simulink model "MicroADAPCPU1"  (R2024a)
settings: Solver=FixedStepAuto  StartTime=0.0  StopTime=Inf  RelTol=1e-3  EnableMultiTasking=on
PreLoadFcn:
  | %Condiciones iniciales
  | id0=single(0);
  | iq0=single(0);
  | w0=single(0);
  | Thetha0=single(0);
  | deltars=0;
  | deltaLd=0;
  | deltaLq=0;
  | deltaphi=0;
  | 
  | %Parametros Axel;
  | Rs=single(1.1); %Ohms
  | L=single(0.00372);
  | Ld=L; %Henrry
  | Lq=L; %Henrry
  | Jm=single(0.00023998); %Kg m2
  | Rm=single(0.0006738); %Nm s
  | rm=Rm;
  | phi=single(0.1099); %Wb
  | %0.0582
  | np=single(8);
values from neighbouring files (symbols this model uses):
  target = mcb_SetProcessorDetails('F28379D',PWM_frequency)    [Para_Motor_Micro.m]
  Ts_com = 2*1*Ts    (= 6e-05)    [Para_Motor_Micro.m]
undefined symbols (not defined in the file or in its folder): C28x, CPU1, CPU2, DiscIntNeverNeededParam, Down, GPTRIP1SEL, GPTRIP2SEL, inverter, PWM_Counter_PeriodVel, TZ1, TZ2, Up
libraries: c2802xlib x12, mcbcontrolslib x9, c2837xDlib x8, simulink x4, mcbpositiondecoderlib x3, c280xlib x3, svdutilitieslib x2, eeTransforms x1, c2000lib x1
(part 2 of 2)

== system MicroADAPCPU1/Comms/SCI (Code Generation) 40khz/While Iterator Subsystem ==
  Data : Inport
  Iteration : Inport  Port=2
  Add : Sum  Inputs=+-  OutDataTypeStr=Inherit: Same as first input
  Index Vector : MultiPortSwitch  Inputs=1  SaturateOnIntegerOverflow=off  InputSameDT=off
  SCI Transmit : c280xlib/SCI Transmit  sciModule=A  dataHead=''  dataTail=''  blockingMode=on  outputStatus=off
  While Iterator : WhileIterator  MaxIters=-1  WhileBlockType=do-while  ShowIterationPort=on  OutputDataType=int16
  wires:
  Iteration/1 -> Add/1
  Add/1 -> While Iterator/1
  Index Vector/1 -> SCI Transmit/1
  Data/1 -> Index Vector/2
  While Iterator/1 -> Index Vector/1, Add/2

== system MicroADAPCPU1/ADC-PWM Subsystem1/Control_System/Clark Transform Filter/Clarke Transformation ==
  Ia : Inport
  Ib : Inport  Port=2
  1 : Constant  Value=0.57735026918963  OutDataTypeStr=Inherit: Inherit via back propagation
  2 : Constant  Value=2  OutDataTypeStr=Inherit: Inherit via back propagation  SampleTime=Inf
  Product : Product  OutDataTypeStr=single
  Product1 : Product  OutDataTypeStr=Inherit: Same as first input
  Sum1 : Sum  Inputs=|++  OutDataTypeStr=Inherit: Same as first input
  Out1 : Outport
  Out2 : Outport  Port=2
  wires:
  Ib/1 -> Product/2
  Ia/1 -> Out1/1, Sum1/1
  Sum1/1 -> Product1/2
  2/1 -> Product/1
  Product1/1 -> Out2/1
  Product/1 -> Sum1/2
  1/1 -> Product1/1

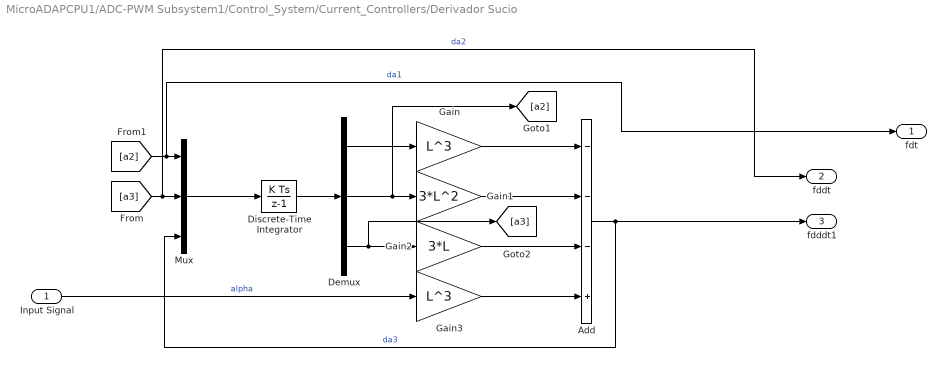
== system MicroADAPCPU1/ADC-PWM Subsystem1/Control_System/Current_Controllers/Derivador Sucio ==
  Input Signal : Inport
  Add : Sum  Inputs=---+
  Demux : Demux  Outputs=3
  Discrete-Time Integrator : DiscreteIntegrator  InitialCondition=[0; 0; 0]  SampleTime=-1  ICPrevOutput=DiscIntNeverNeededParam  ICPrevScaledInput=DiscIntNeverNeededParam
  Gain : Gain  Gain=L^3  OutDataTypeStr=double
  Gain1 : Gain  Gain=3*L^2  OutDataTypeStr=double
  Gain2 : Gain  Gain=3*L  OutDataTypeStr=double
  Gain3 : Gain  Gain=L^3  OutDataTypeStr=double
  Mux : Mux  Inputs=3
  fdt : Outport
  fddt : Outport  Port=2
  fdddt1 : Outport  Port=3
  wires:
  Demux/1 -> Gain/1
  Gain3/1 -> Add/4
  Input Signal/1 -> Gain3/1  "alpha"
  Demux/2 -> [a2], Gain1/1
  Gain2/1 -> Add/3
  Gain1/1 -> Add/2
  Gain/1 -> Add/1
  Demux/3 -> [a3], Gain2/1
  Add/1 -> fdddt1/1, Mux/3  "da3"
  [a3] -> Mux/2, fddt/1  "da2"
  [a2] -> fdt/1, Mux/1  "da1"
  Discrete-Time Integrator/1 -> Demux/1
  Mux/1 -> Discrete-Time Integrator/1

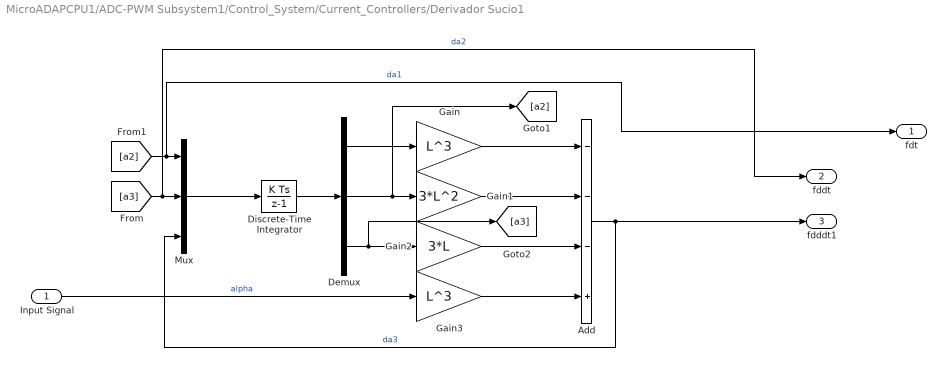
== system MicroADAPCPU1/ADC-PWM Subsystem1/Control_System/Current_Controllers/Derivador Sucio1 ==
  Input Signal : Inport
  Add : Sum  Inputs=---+
  Demux : Demux  Outputs=3
  Discrete-Time Integrator : DiscreteIntegrator  InitialCondition=[0; 0; 0]  SampleTime=-1  ICPrevOutput=DiscIntNeverNeededParam  ICPrevScaledInput=DiscIntNeverNeededParam
  Gain : Gain  Gain=L^3  OutDataTypeStr=double
  Gain1 : Gain  Gain=3*L^2  OutDataTypeStr=double
  Gain2 : Gain  Gain=3*L  OutDataTypeStr=double
  Gain3 : Gain  Gain=L^3  OutDataTypeStr=double
  Mux : Mux  Inputs=3
  fdt : Outport
  fddt : Outport  Port=2
  fdddt1 : Outport  Port=3
  wires:
  Demux/1 -> Gain/1
  Gain3/1 -> Add/4
  Input Signal/1 -> Gain3/1  "alpha"
  Demux/2 -> [a2], Gain1/1
  Gain2/1 -> Add/3
  Gain1/1 -> Add/2
  Gain/1 -> Add/1
  Demux/3 -> [a3], Gain2/1
  Add/1 -> fdddt1/1, Mux/3  "da3"
  [a3] -> Mux/2, fddt/1  "da2"
  [a2] -> fdt/1, Mux/1  "da1"
  Discrete-Time Integrator/1 -> Demux/1
  Mux/1 -> Discrete-Time Integrator/1

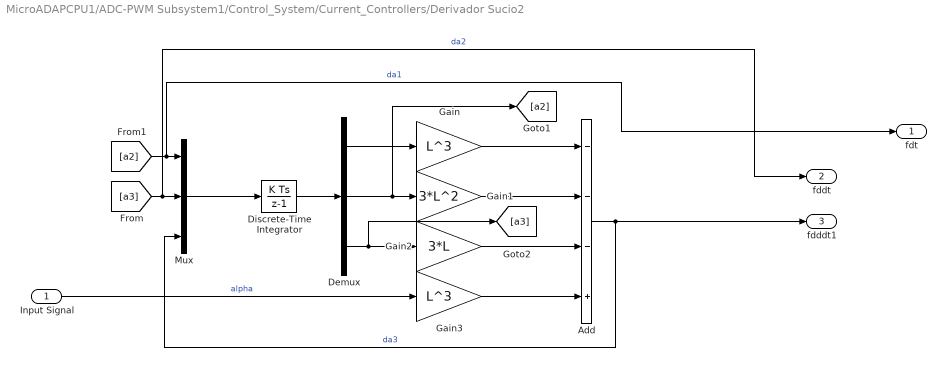
== system MicroADAPCPU1/ADC-PWM Subsystem1/Control_System/Current_Controllers/Derivador Sucio2 ==
  Input Signal : Inport
  Add : Sum  Inputs=---+
  Demux : Demux  Outputs=3
  Discrete-Time Integrator : DiscreteIntegrator  InitialCondition=[0; 0; 0]  SampleTime=-1  ICPrevOutput=DiscIntNeverNeededParam  ICPrevScaledInput=DiscIntNeverNeededParam
  Gain : Gain  Gain=L^3  OutDataTypeStr=double
  Gain1 : Gain  Gain=3*L^2  OutDataTypeStr=double
  Gain2 : Gain  Gain=3*L  OutDataTypeStr=double
  Gain3 : Gain  Gain=L^3  OutDataTypeStr=double
  Mux : Mux  Inputs=3
  fdt : Outport
  fddt : Outport  Port=2
  fdddt1 : Outport  Port=3
  wires:
  Demux/1 -> Gain/1
  Gain3/1 -> Add/4
  Input Signal/1 -> Gain3/1  "alpha"
  Demux/2 -> [a2], Gain1/1
  Gain2/1 -> Add/3
  Gain1/1 -> Add/2
  Gain/1 -> Add/1
  Demux/3 -> [a3], Gain2/1
  Add/1 -> fdddt1/1, Mux/3  "da3"
  [a3] -> Mux/2, fddt/1  "da2"
  [a2] -> fdt/1, Mux/1  "da1"
  Discrete-Time Integrator/1 -> Demux/1
  Mux/1 -> Discrete-Time Integrator/1

== system MicroADAPCPU1/ADC-PWM Subsystem1/Mesurments/Position Mesurment/IndexFinder ==
  In1 : Inport
  Enable : EnablePort
  AND : Logic  AllPortsSameDT=off  OutDataTypeStr=boolean
  Compare To Constant : simulink/Logic and Bit Operations/Compare To Constant  relop===  const=0  OutDataTypeStr=boolean
  Compare To Constant1 : simulink/Logic and Bit Operations/Compare To Constant  relop=>  const=0  OutDataTypeStr=boolean
  Delay3 : Delay  DelayLength=1
  EnClosedLoop : Outport
  wires:
  In1/1 -> Delay3/1, Compare To Constant1/1
  Compare To Constant1/1 -> AND/2
  Compare To Constant/1 -> AND/1
  Delay3/1 -> Compare To Constant/1
  AND/1 -> EnClosedLoop/1

== system MicroADAPCPU1/Comms/Comms/SCI (Serial Comunication)/Data_Logging ==
  note: Fast Serial Data Monitoring (32-bit)
  Data_Log : Inport
  Counter Limited : simulink/Sources/Counter Limited  uplimit=600-1  tsamp=-1
  Data : Subsystem  TreatAsAtomicUnit=on
  End : Subsystem  TreatAsAtomicUnit=on
  If : If  IfExpression=u1 == 0  ElseIfExpressions=u1 == 599
  Merge : Merge  Inputs=3
  Merge1 : Merge  Inputs=3
  Mux : Mux  Inputs=2
  Start : Subsystem  TreatAsAtomicUnit=on
  Width : Width  OutDataTypeMode=All ports same datatype  DataType=uint16
  SCI_Tx : Outport
  wires:
  If/3 -> Data/Action
  Data/1(Data_out) -> Merge/3
  Width/1 -> Data/2(Data_width), End/2(Data_width), Start/2(Data_width)
  Merge/1 -> Mux/1  "SCI_Tx_Data"
  Counter Limited/1 -> If/1
  Start/2(Iteration) -> Merge1/1
  Start/1(Data_out) -> Merge/1
  If/2 -> End/Action
  Merge1/1 -> Mux/2  "SCI_Tx_Iteration"
  If/1 -> Start/Action
  End/1(Data_out) -> Merge/2
  End/2(Iteration) -> Merge1/2
  Data/2(Iteration) -> Merge1/3
  Mux/1 -> SCI_Tx/1
  Data_Log/1 -> Width/1, Start/1(Data), End/1(Data), Data/1(Data)

== system MicroADAPCPU1/Comms/Comms/SCI (Serial Comunication)/While Iterator Subsystem ==
  Data : Inport
  Iteration : Inport  Port=2
  Add : Sum  Inputs=+-  OutDataTypeStr=Inherit: Same as first input
  Index Vector : MultiPortSwitch  Inputs=1  SaturateOnIntegerOverflow=off  InputSameDT=off
  SCI Transmit : c280xlib/SCI Transmit  sciModule=A  dataHead=''  dataTail=''  frameSize=1  blockingMode=on  outputStatus=off
  While Iterator : WhileIterator  MaxIters=-1  WhileBlockType=do-while  ShowIterationPort=on  OutputDataType=int16
  wires:
  While Iterator/1 -> Add/2, Index Vector/1
  Data/1 -> Index Vector/2
  Index Vector/1 -> SCI Transmit/1
  Add/1 -> While Iterator/1
  Iteration/1 -> Add/1

== system MicroADAPCPU1/Comms/SCI (Code Generation) 40khz/Data_Logging/Data ==
  Data : Inport
  Data_width : Inport  Port=2
  Action Port : ActionPort
  Dummy : Constant  Value=hex2dec('0000')  OutDataTypeStr=uint32
  Mux : Mux  Inputs=2
  Data_out : Outport  VectorParamsAs1DForOutWhenUnconnected=off
  Iteration : Outport  Port=2  VectorParamsAs1DForOutWhenUnconnected=off
  wires:
  Mux/1 -> Data_out/1
  Dummy/1 -> Mux/2
  Data/1 -> Mux/1
  Data_width/1 -> Iteration/1

== system MicroADAPCPU1/Comms/SCI (Code Generation) 40khz/Data_Logging/End ==
  Data : Inport
  Data_width : Inport  Port=2
  Action Port : ActionPort
  Bias : Bias  Bias=1  SaturateOnIntegerOverflow=off
  End : Constant  Value=hex2dec('45454545')  OutDataTypeStr=uint32
  Mux : Mux  Inputs=2
  Data_out : Outport  VectorParamsAs1DForOutWhenUnconnected=off
  Iteration : Outport  Port=2  VectorParamsAs1DForOutWhenUnconnected=off
  wires:
  Mux/1 -> Data_out/1
  End/1 -> Mux/2
  Bias/1 -> Iteration/1
  Data_width/1 -> Bias/1
  Data/1 -> Mux/1

== system MicroADAPCPU1/Comms/SCI (Code Generation) 40khz/Data_Logging/Start ==
  Data : Inport
  Data_width : Inport  Port=2
  Action Port : ActionPort
  Bias : Bias  Bias=1  SaturateOnIntegerOverflow=off
  Mux : Mux  Inputs=2
  Start : Constant  Value=hex2dec('53535353')  OutDataTypeStr=uint32
  Data_out : Outport  VectorParamsAs1DForOutWhenUnconnected=off
  Iteration : Outport  Port=2  VectorParamsAs1DForOutWhenUnconnected=off
  wires:
  Mux/1 -> Data_out/1
  Start/1 -> Mux/1
  Bias/1 -> Iteration/1
  Data_width/1 -> Bias/1
  Data/1 -> Mux/2

== system MicroADAPCPU1/Comms/Comms/SCI (Serial Comunication)/Data_Logging/Data ==
  Data : Inport
  Data_width : Inport  Port=2
  Action Port : ActionPort  ActionPortLabel=else
  Dummy : Constant  Value=hex2dec('0000')  OutDataTypeStr=uint32
  Mux : Mux  Inputs=2
  Data_out : Outport  VectorParamsAs1DForOutWhenUnconnected=off
  Iteration : Outport  Port=2  VectorParamsAs1DForOutWhenUnconnected=off
  wires:
  Data_width/1 -> Iteration/1
  Data/1 -> Mux/1
  Dummy/1 -> Mux/2
  Mux/1 -> Data_out/1

== system MicroADAPCPU1/Comms/Comms/SCI (Serial Comunication)/Data_Logging/End ==
  Data : Inport
  Data_width : Inport  Port=2
  Action Port : ActionPort  ActionPortLabel=elseif(u1 == 599)
  Bias : Bias  Bias=1  SaturateOnIntegerOverflow=off
  End : Constant  Value=hex2dec('45454545')  OutDataTypeStr=uint32
  Mux : Mux  Inputs=2
  Data_out : Outport  VectorParamsAs1DForOutWhenUnconnected=off
  Iteration : Outport  Port=2  VectorParamsAs1DForOutWhenUnconnected=off
  wires:
  Data/1 -> Mux/1
  Data_width/1 -> Bias/1
  Bias/1 -> Iteration/1
  End/1 -> Mux/2
  Mux/1 -> Data_out/1

== system MicroADAPCPU1/Comms/Comms/SCI (Serial Comunication)/Data_Logging/Start ==
  Data : Inport
  Data_width : Inport  Port=2
  Action Port : ActionPort  ActionPortLabel=if(u1 == 0)
  Bias : Bias  Bias=1  SaturateOnIntegerOverflow=off
  Mux : Mux  Inputs=2
  Start : Constant  Value=hex2dec('53535353')  OutDataTypeStr=uint32
  Data_out : Outport  VectorParamsAs1DForOutWhenUnconnected=off
  Iteration : Outport  Port=2  VectorParamsAs1DForOutWhenUnconnected=off
  wires:
  Data/1 -> Mux/2
  Data_width/1 -> Bias/1
  Bias/1 -> Iteration/1
  Start/1 -> Mux/1
  Mux/1 -> Data_out/1

== matlab function MicroADAPCPU1/ADC-PWM Subsystem1/Control_System/Current_Controllers/Control  ==
  data: Ted input; id input; iq input; id_d output; iq_d output; u output; w input; did input; diq input; diq_d input; phi parameter; Ld parameter; Lq parameter; Rs parameter; np parameter; theta input; v output; u_total output; Theta_tilde_p output
function [id_d, iq_d, u, v, u_total, Theta_tilde_p] = fcn(Ted, id, iq, w, did, diq, diq_d, phi, Ld, Lq, Rs, np, theta)
%function [id_d, iq_d, u] = fcn(Ted, id, iq, w, diq_d, phi, Ld, Lq, Rs, np)

%--Deseadas 

iq_d=single(Ted*(1/(np*0.1099))); 
id_d=single(0);%-phi/(2*(Ld-Lq))-sqrt(phi^2/(4*(Ld-Lq)^2)+iq_d^2);
did_d=single(0); %-iq_d*(phi/(4*(Ld-Lq)^2)+iq_d^2)^(-1/2);
% 
% Phi=single([0; phi]);
% Q=single([Ld 0; 0 Lq]); 
% Qinv=single([1/Ld 0; 0 1/Lq]);
% J=single([0 -1; 1 0]);
% 
% x=single([id_d; iq_d]);
% xp=single([did_d; diq_d]);
% 
% ud=single(Q*(xp+Rs*Qinv*x+np*w*Qinv*J*Q*x+np*w*Qinv*Phi));
% 
% 
% ud_d=single(ud(1));
% uq_d=single(ud(2));
ud_d=single(Ld*did_d+Rs*id_d-np*w*Lq*iq_d);
uq_d=single(Lq*diq_d+Rs*iq_d+np*w*phi+np*w*Ld*id_d);

%--Control Nominal
% 
% e1=single(id-id_d);
% e2=single(iq-iq_d);

ed=id-id_d;
eq=iq-iq_d;

e=single([ed; eq]);

%Ganancias 
k1=single(100);
k2=single(100);


% utilde=single(-K*e+np*w*J*Q*e);
% 
% udtilde=single(utilde(1));
% uqtilde=single(utilde(2));
% 


udtilde=single(-k1*ed-np*w*Lq*eq);
uqtilde=single(-k2*eq+np*w*Ld*ed);

 % ud=udtilde+ud_d;
 % uq=uqtilde+uq_d;
ud=single(udtilde+ud_d);
uq=single(uqtilde+uq_d);

u=single([ud; uq]);

%Contorl Adaptable
gama=single(0.01);

gamma1=single(gama);
gamma2=single(gama); 
gamma3=single(gama);
gamma4=single(gama); 

dTheta_1=single(gamma1*(id*ed+iq*eq));
dTheta_2=single(gamma2*(did*ed+np*w*iq*eq));
dTheta_3=single(gamma3*(-np*w*iq*ed+diq*eq));
dTheta_4=single(gamma4*np*w*eq);

Theta_tilde_p=single([dTheta_1; dTheta_2; dTheta_3; dTheta_4]);


vd=single(id*theta(1)+did*theta(2)-np*w*iq*theta(3));
vq=single(iq*theta(1)+np*w*id*theta(2)+diq*theta(3)+np*w*theta(4));


v=single([vd;vq]);

u_total=single(u-v);

== matlab function MicroADAPCPU1/ADC-PWM Subsystem1/Mesurments/Voltage Mesurment/Pole to phase 1 ==
  data: Vag input; Vn output; Vbg input; Vcg input

function Vn  = fcn(Vag,Vbg,Vcg)
% Vg=[Vag;Vbg;Vcg];
% Vn=[2/3,-1/3,-1/3;-1/3,2/3,-1/3;-1/3,-1/3,2/3]*Vg;
% 
 Van=single(2/3*Vag-1/3*Vbg -1/3*Vcg) ;
 Vbn=single(2/3*Vbg-1/3*Vag -1/3*Vcg) ;
 Vcn=single(2/3*Vcg-1/3*Vbg -1/3*Vag) ;
Vn=[Van;Vbn;Vcn];
end
